simulink model "TransmissionController"  (R2026a)
settings: Solver=FixedStepAuto  StopTime=65  FixedStep=0.5
undefined symbols (not defined in the file): previousGear, previousPark, rangeSelection, vehicleSpeed
libraries: simulink x3, sl_discontinuities x1
settings Model: DataDictionary=ETRS_data.sldd  Creator=macec  LastModifiedBy=burat
settings RTWCC: Toolchain=MinGW64 | gmake (64-bit Windows)

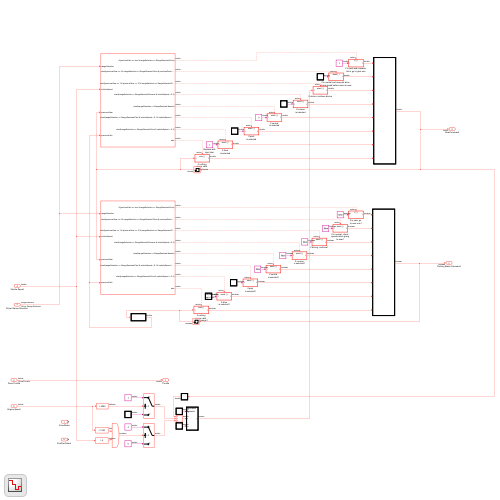
[thumbnail: Simulink's stored preview of the top-level diagram]
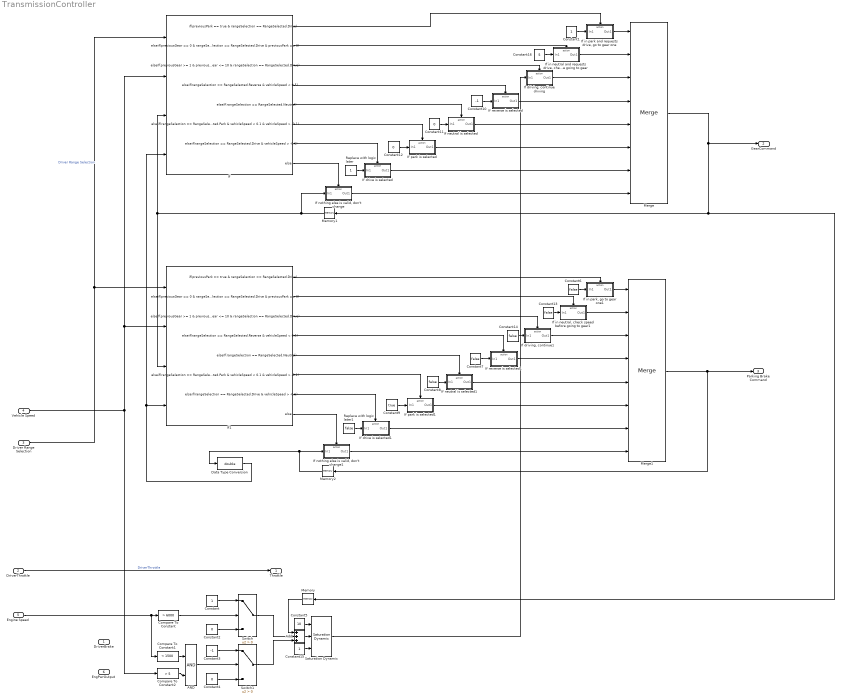
== system TransmissionController ==
  DriverBrake : Inport  OutDataTypeStr=double  PortDimensions=1
  DriverThrottle : Inport  Port=2  OutDataTypeStr=double  PortDimensions=1
  Driver Range Selection : Inport  Port=3  OutDataTypeStr=Enum: RangeSelected  PortDimensions=1  Interpolate=off
  Vehicle Speed : Inport  Port=4  OutDataTypeStr=double  PortDimensions=1
  Engine Speed : Inport  Port=5  OutDataTypeStr=double  PortDimensions=1
  EngPwrOutput : Inport  Port=6
  AND : Logic  IconShape=distinctive  AllPortsSameDT=off  OutDataTypeStr=boolean
  Add : Sum  Inputs=+++
  Compare To Constant : simulink/Logic and Bit Operations/Compare To Constant  relop=>  const=6000  OutDataTypeStr=boolean
  Compare To Constant1 : simulink/Logic and Bit Operations/Compare To Constant  relop=<  const=1500  OutDataTypeStr=boolean
  Compare To Constant2 : simulink/Logic and Bit Operations/Compare To Constant  relop=>  const=5  OutDataTypeStr=boolean
  Constant : Constant
  Constant1 : Constant
  Constant10 : Constant  Value=-1
  Constant{2,4,11..12} (4 alike) : Constant  Value=0
  Constant{6..8,13..14} (5 alike) : Constant  Value=false
  Constant15 : Constant
  Constant16 : Constant  Value=5
  Constant3 : Constant  Value=-1
  Constant5 : Constant  Value=10
  Constant9 : Constant  Value=true
  Data Type Conversion : DataTypeConversion  OutDataTypeStr=double  SaturateOnIntegerOverflow=off  RndMeth=Floor
  If : If  NumInputs=4  IfExpression=previousPark == true & rangeSelection == RangeSelected.Drive  ElseIfExpressions=previousGear == 0 & rangeSelection == RangeSelected.Drive & previousPark == 0,previousGear >= 1 & previousGear <= 10 & rangeSelection == RangeSelected.Drive,rangeSelection == RangeSelected.Reverse & vehicleSpeed < 0.5,rangeSelection == RangeSelected.Neutral,rangeSelection == RangeSelected.Park & vehicleSpeed < 0.1 & vehicleSpeed > -0.1,rangeSelection == RangeSelected.Drive & vehicleSpeed > -0.5  InportLabels=rangeSelection,vehicleSpeed,previousGear,previousPark
  If drive is selected : Subsystem  TreatAsAtomicUnit=on
  If drive is selected1 : Subsystem  TreatAsAtomicUnit=on
  "If driving, continue driving" : Subsystem  TreatAsAtomicUnit=on
  "If driving, continue1" : Subsystem  TreatAsAtomicUnit=on
  "If in neutral and requests drive, check speed before going to gear" : Subsystem  TreatAsAtomicUnit=on
  "If in neutral, check speed before going to gear1" : Subsystem  TreatAsAtomicUnit=on
  "If in park and requests drive, go to gear one" : Subsystem  TreatAsAtomicUnit=on
  "If in park, go to gear one1" : Subsystem  TreatAsAtomicUnit=on
  If neutral is selected : Subsystem  TreatAsAtomicUnit=on
  If neutral is selected1 : Subsystem  TreatAsAtomicUnit=on
  "If nothing else is valid, don't change" : Subsystem  TreatAsAtomicUnit=on
  "If nothing else is valid, don't change1" : Subsystem  TreatAsAtomicUnit=on
  If park is selected : Subsystem  TreatAsAtomicUnit=on
  If park is selected1 : Subsystem  TreatAsAtomicUnit=on
  If reverse is selected : Subsystem  TreatAsAtomicUnit=on
  If reverse is selected1 : Subsystem  TreatAsAtomicUnit=on
  If1 : If  NumInputs=4  IfExpression=previousPark == true & rangeSelection == RangeSelected.Drive  ElseIfExpressions=previousGear == 0 & rangeSelection == RangeSelected.Drive & previousPark == 0,previousGear >= 1 & previousGear <= 10 & rangeSelection == RangeSelected.Drive,rangeSelection == RangeSelected.Reverse & vehicleSpeed < 0.5,rangeSelection == RangeSelected.Neutral,rangeSelection == RangeSelected.Park & vehicleSpeed < 0.1 & vehicleSpeed > -0.1,rangeSelection == RangeSelected.Drive & vehicleSpeed > -0.5  InportLabels=rangeSelection,vehicleSpeed,previousGear,previousPark
  Memory : Memory  InheritSampleTime=on
  Memory1 : Memory  InheritSampleTime=on
  Memory2 : Memory  InheritSampleTime=on
  Merge : Merge  Inputs=8
  Merge1 : Merge  Inputs=8
  Replace with logic later : Constant
  Replace with logic later1 : Constant  Value=false
  Saturation Dynamic : sl_discontinuities/Saturation Dynamic  OutMin=[]  OutMax=[]  OutDataTypeStr=Inherit: Same as second input  OutDataType=fixdt(1, 16)  OutScaling=2^-10  DoSatur=off
      settings: LibrarySourceBlock=|
      | simulink/Discontinuities/Saturation
      | Dynamic
  Switch : Switch  Criteria=u2 > Threshold  SaturateOnIntegerOverflow=off  InputSameDT=off
  Switch1 : Switch  Criteria=u2 > Threshold  SaturateOnIntegerOverflow=off  InputSameDT=off
  Throttle : Outport  OutDataTypeStr=double  PortDimensions=1
  GearCommand : Outport  Port=2  OutDataTypeStr=double  PortDimensions=1
  Parking Brake Command : Outport  Port=3  OutDataTypeStr=boolean  PortDimensions=1
  wires:
  Driver Range Selection/1 -> If1/1, If/1  "Driver Range Selection"
  Vehicle Speed/1 -> If1/2, If/2, Compare To Constant2/1
  Engine Speed/1 -> Compare To Constant/1, Compare To Constant1/1
  Compare To Constant/1 -> Switch/2
  Constant/1 -> Switch/1
  Constant2/1 -> Switch/3
  Constant3/1 -> Switch1/1
  Constant4/1 -> Switch1/3
  Compare To Constant2/1 -> AND/2
  AND/1 -> Switch1/2
  Compare To Constant1/1 -> AND/1
  Switch1/1 -> Add/3
  Switch/1 -> Add/2
  Memory/1 -> Add/1
  Constant5/1 -> Saturation Dynamic/1
  Add/1 -> Saturation Dynamic/2
  DriverThrottle/1 -> Throttle/1  "DriverThrottle"
  If/4 -> If reverse is selected/Action
  Merge/1 -> Memory/1, Memory1/1, GearCommand/1
  Constant10/1 -> If reverse is selected/1(In1)
  If reverse is selected/1(Out1) -> Merge/4
  Constant11/1 -> If neutral is selected/1(In1)
  If neutral is selected/1(Out1) -> Merge/5
  If/5 -> If neutral is selected/Action
  If/6 -> If park is selected/Action
  Constant12/1 -> If park is selected/1(In1)
  If park is selected/1(Out1) -> Merge/6
  Replace with logic later/1 -> If drive is selected/1(In1)
  If drive is selected/1(Out1) -> Merge/7
  "If nothing else is valid, don't change"/1(Out1) -> Merge/8
  Memory1/1 -> If1/3, If/3, "If nothing else is valid, don't change"/1(In1)
  If/1 -> "If in park and requests drive, go to gear one"/Action
  Constant1/1 -> "If in park and requests drive, go to gear one"/1(In1)
  If/2 -> "If in neutral and requests drive, check speed before going to gear"/Action
  If/3 -> "If driving, continue driving"/Action
  "If in park and requests drive, go to gear one"/1(Out1) -> Merge/1
  "If in neutral and requests drive, check speed before going to gear"/1(Out1) -> Merge/2
  "If driving, continue driving"/1(Out1) -> Merge/3
  Constant6/1 -> "If in park, go to gear one1"/1(In1)
  "If in park, go to gear one1"/1(Out1) -> Merge1/1
  "If driving, continue1"/1(Out1) -> Merge1/3
  If1/3 -> "If driving, continue1"/Action
  If neutral is selected1/1(Out1) -> Merge1/5
  If1/2 -> "If in neutral, check speed before going to gear1"/Action
  If park is selected1/1(Out1) -> Merge1/6
  If drive is selected1/1(Out1) -> Merge1/7
  "If nothing else is valid, don't change1"/1(Out1) -> Merge1/8
  Constant9/1 -> If park is selected1/1(In1)
  If1/1 -> "If in park, go to gear one1"/Action
  "If in neutral, check speed before going to gear1"/1(Out1) -> Merge1/2
  Constant7/1 -> If reverse is selected1/1(In1)
  If1/6 -> If park is selected1/Action
  Replace with logic later1/1 -> If drive is selected1/1(In1)
  If1/7 -> If drive is selected1/Action
  If1/4 -> If reverse is selected1/Action
  Memory2/1 -> "If nothing else is valid, don't change1"/1(In1), Data Type Conversion/1
  Constant8/1 -> If neutral is selected1/1(In1)
  If1/5 -> If neutral is selected1/Action
  If1/8 -> "If nothing else is valid, don't change1"/Action
  Merge1/1 -> Parking Brake Command/1, Memory2/1
  If reverse is selected1/1(Out1) -> Merge1/4
  Constant13/1 -> "If in neutral, check speed before going to gear1"/1(In1)
  Constant14/1 -> "If driving, continue1"/1(In1)
  Saturation Dynamic/1 -> "If driving, continue driving"/1(In1)
  Constant16/1 -> "If in neutral and requests drive, check speed before going to gear"/1(In1)
  Data Type Conversion/1 -> If/4, If1/4
  Constant15/1 -> Saturation Dynamic/3
  If/7 -> If drive is selected/Action
  If/8 -> "If nothing else is valid, don't change"/Action

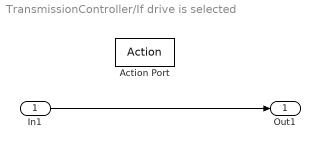
== system TransmissionController/If drive is selected ==
  In1 : Inport
  Action Port : ActionPort  ActionPortLabel=elseif(rangeSelection == RangeSelected.Drive & vehicleSpeed > -0.5)
  Out1 : Outport
  wires:
  In1/1 -> Out1/1

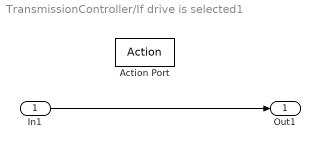
== system TransmissionController/If drive is selected1 ==
  In1 : Inport
  Action Port : ActionPort  ActionPortLabel=elseif(rangeSelection == RangeSelected.Drive & vehicleSpeed > -0.5)
  Out1 : Outport
  wires:
  In1/1 -> Out1/1

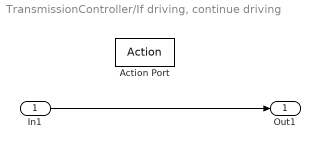
== system TransmissionController/If driving, continue driving ==
  In1 : Inport
  Action Port : ActionPort  ActionPortLabel=elseif(previousGear >= 1 & previousGear <= 10 & rangeSelection == RangeSelected.Drive)
  Out1 : Outport
  wires:
  In1/1 -> Out1/1

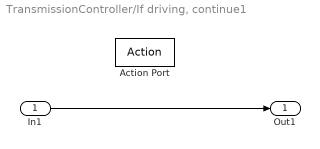
== system TransmissionController/If driving, continue1 ==
  In1 : Inport
  Action Port : ActionPort  ActionPortLabel=elseif(previousGear >= 1 & previousGear <= 10 & rangeSelection == RangeSelected.Drive)
  Out1 : Outport
  wires:
  In1/1 -> Out1/1

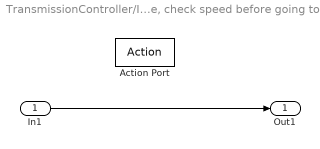
== system TransmissionController/If in neutral and requests drive, check speed before going to gear ==
  In1 : Inport
  Action Port : ActionPort  ActionPortLabel=elseif(previousGear == 0 & rangeSelection == RangeSelected.Drive & previousPark == 0)
  Out1 : Outport
  wires:
  In1/1 -> Out1/1

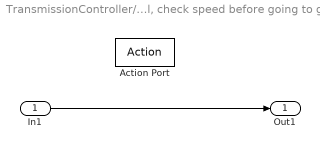
== system TransmissionController/If in neutral, check speed before going to gear1 ==
  In1 : Inport
  Action Port : ActionPort  ActionPortLabel=elseif(previousGear == 0 & rangeSelection == RangeSelected.Drive & previousPark == 0)
  Out1 : Outport
  wires:
  In1/1 -> Out1/1

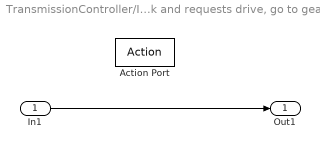
== system TransmissionController/If in park and requests drive, go to gear one ==
  In1 : Inport
  Action Port : ActionPort  ActionPortLabel=if(previousPark == true & rangeSelection == RangeSelected.Drive)
  Out1 : Outport
  wires:
  In1/1 -> Out1/1

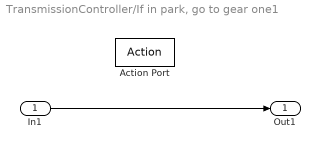
== system TransmissionController/If in park, go to gear one1 ==
  In1 : Inport
  Action Port : ActionPort  ActionPortLabel=if(previousPark == true & rangeSelection == RangeSelected.Drive)
  Out1 : Outport
  wires:
  In1/1 -> Out1/1

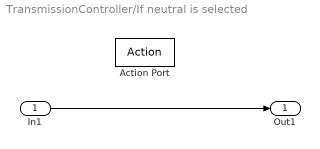
== system TransmissionController/If neutral is selected ==
  In1 : Inport
  Action Port : ActionPort  ActionPortLabel=elseif(rangeSelection == RangeSelected.Neutral)
  Out1 : Outport
  wires:
  In1/1 -> Out1/1

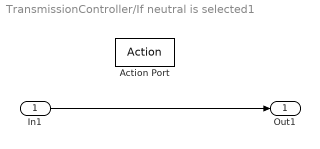
== system TransmissionController/If neutral is selected1 ==
  In1 : Inport
  Action Port : ActionPort  ActionPortLabel=elseif(rangeSelection == RangeSelected.Neutral)
  Out1 : Outport
  wires:
  In1/1 -> Out1/1

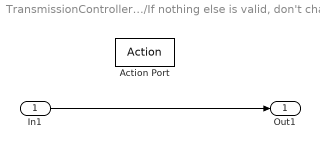
== system TransmissionController/If nothing else is valid, don't change ==
  In1 : Inport
  Action Port : ActionPort  ActionPortLabel=else
  Out1 : Outport
  wires:
  In1/1 -> Out1/1

== system TransmissionController/If nothing else is valid, don't change1 ==
  In1 : Inport
  Action Port : ActionPort  ActionPortLabel=else
  Out1 : Outport
  wires:
  In1/1 -> Out1/1

== system TransmissionController/If park is selected ==
  In1 : Inport
  Action Port : ActionPort  ActionPortLabel=elseif(rangeSelection == RangeSelected.Park & vehicleSpeed < 0.1 & vehicleSpeed > -0.1)
  Out1 : Outport
  wires:
  In1/1 -> Out1/1

== system TransmissionController/If park is selected1 ==
  In1 : Inport
  Action Port : ActionPort  ActionPortLabel=elseif(rangeSelection == RangeSelected.Park & vehicleSpeed < 0.1 & vehicleSpeed > -0.1)
  Out1 : Outport
  wires:
  In1/1 -> Out1/1

== system TransmissionController/If reverse is selected ==
  In1 : Inport
  Action Port : ActionPort  ActionPortLabel=elseif(rangeSelection == RangeSelected.Reverse & vehicleSpeed < 0.5)
  Out1 : Outport
  wires:
  In1/1 -> Out1/1

== system TransmissionController/If reverse is selected1 ==
  In1 : Inport
  Action Port : ActionPort  ActionPortLabel=elseif(rangeSelection == RangeSelected.Reverse & vehicleSpeed < 0.5)
  Out1 : Outport
  wires:
  In1/1 -> Out1/1
